simulink model "PRC_Sleep_u"  (R2015a)
settings: Solver=ode3  StartTime=0.0  StopTime=3000  FixedStep=0.01  RelTol=1e-5
undefined symbols (not defined in the file): D, f, H0, T, theta0, umax
settings Model: Creator=Zhang Jiaxiang  LastModifiedBy=Jiawei Yin
settings DataIOCC: LimitDataPoints=off  SignalLoggingSaveFormat=ModelDataLogs
settings OptimizationCC: ExpressionDepthLimit=2147483647
settings DebuggingCC: UnderspecifiedInitializationDetection=Classic  MergeDetectMultiDrivingBlocksExec=none  FcnCallInpInsideContextMsg=UseLocalSettings  StateNameClashWarn=warning
settings GRTTargetCC: CombineOutputUpdateFcns=off  GRTInterface=on

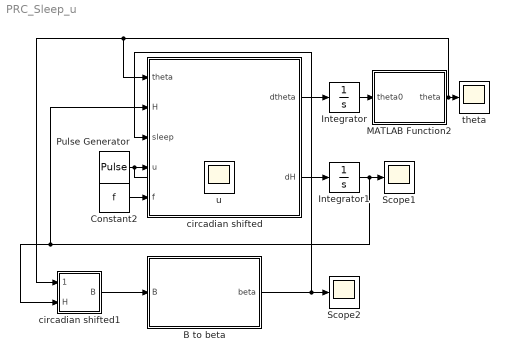
== system PRC_Sleep_u ==
  "B to beta " : Subsystem
  Constant2 : Constant  Value=f
  Integrator : Integrator  InitialCondition=theta0
  Integrator1 : Integrator  InitialCondition=H0
  MATLAB Function2 : MATLAB Function  TreatAsAtomicUnit=on
      settings: PermitHierarchicalResolution=ParametersOnly
  Pulse Generator : DiscretePulseGenerator  PulseType=Time based  Amplitude=umax  Period=T  PulseWidth=D
  Scope1 : Scope
      settings: TimeRange=auto  MaxDataPoints=1000000  SaveName=H  YMin=-0.03001  YMax=0.84118  SampleTime=-1  DataFormat=Array
  Scope2 : Scope
      settings: TimeRange=auto  MaxDataPoints=100000000  SaveName=sleep  YMin=-0.125  YMax=1.125  SampleTime=-1  DataFormat=Array
  circadian shifted : MATLAB Function  TreatAsAtomicUnit=on
      settings: PermitHierarchicalResolution=ParametersOnly
  circadian shifted1 : MATLAB Function  TreatAsAtomicUnit=on
      settings: PermitHierarchicalResolution=ParametersOnly
  theta : Scope
      settings: TimeRange=auto  MaxDataPoints=1000000  SaveName=theta  YMin=-0.78539  YMax=7.06847  SampleTime=-1  DataFormat=Array
  u : Scope
      settings: TimeRange=auto  MaxDataPoints=1000000  SaveName=u  YMin=-0.03001  YMax=0.84118  SampleTime=-1  DataFormat=Array
  wires:
  circadian shifted/1(dtheta) -> Integrator/1
  circadian shifted/2(dH) -> Integrator1/1
  Integrator1/1 -> Scope1/1, circadian shifted1/2(H), circadian shifted/2(H)
  Pulse Generator/1 -> u/1, circadian shifted/4(u)
  Constant2/1 -> circadian shifted/5(f)
  circadian shifted1/1(B) -> "B to beta "/1(B)
  "B to beta "/1(beta) -> Scope2/1, circadian shifted/3(sleep)
  Integrator/1 -> MATLAB Function2/1(theta0)
  MATLAB Function2/1(theta) -> circadian shifted1/1(theta), circadian shifted/1(theta), theta/1

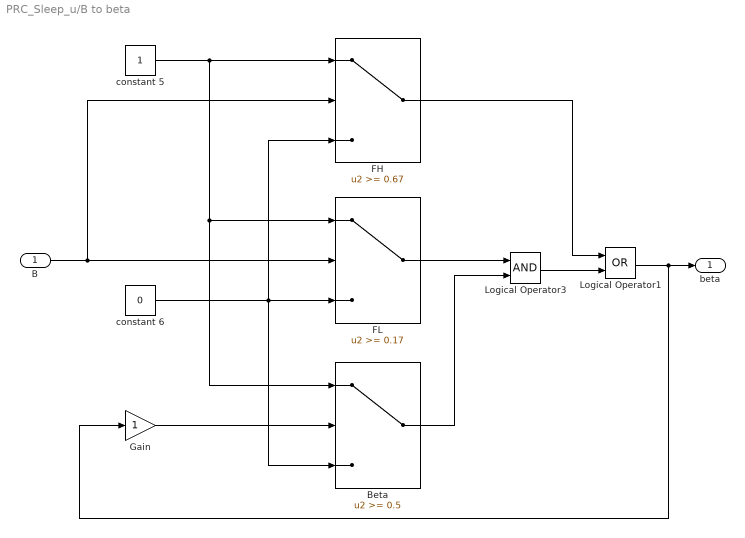
== system PRC_Sleep_u/B to beta  ==
  B : Inport
  Beta : Switch  Threshold=0.5
  FH : Switch  Threshold=0.67
  FL : Switch  Threshold=0.17
  Gain : Gain
  Logical Operator1 : Logic  Operator=OR  AllPortsSameDT=off  OutDataTypeStr=boolean
  Logical Operator3 : Logic  AllPortsSameDT=off  OutDataTypeStr=boolean
  constant 5 : Constant
  constant 6 : Constant  Value=0
  beta : Outport
  wires:
  constant 5/1 -> Beta/1, FL/1, FH/1
  constant 6/1 -> Beta/3, FH/3, FL/3
  B/1 -> FH/2, FL/2
  Logical Operator1/1 -> Gain/1, beta/1
  Gain/1 -> Beta/2
  FL/1 -> Logical Operator3/1
  Beta/1 -> Logical Operator3/2
  Logical Operator3/1 -> Logical Operator1/2
  FH/1 -> Logical Operator1/1

== matlab function PRC_Sleep_u/circadian shifted ==
  data: theta input; H input; sleep input; u input; dtheta output; dH output; f input
function [ dtheta,dH] = fcn(theta,H,sleep,u,f)
%#eml
omega0=2*pi/24.2;
tr=18.2;
td=4.2;
dtheta=omega0+interp1q(f(:,1),f(:,2),theta)*(1-sleep)*u;
dH=(1-H)*(1-sleep)/tr-H*sleep/td;

== matlab function PRC_Sleep_u/circadian shifted1 ==
  data: theta input; H input; B output
function B = fcn(theta,H)
%#eml
B=H-0.1333*cos(theta);

== matlab function PRC_Sleep_u/MATLAB Function2 ==
  data: theta0 input; theta output
function theta  = fcn(theta0)

theta=mod(theta0,2*pi);
